simulink model "iface"  (R2018b)
settings: Solver=FixedStepDiscrete  StartTime=0.0  StopTime=10.0  RelTol=1e-3
settings Model: Creator=matlab  LastModifiedBy=matlab

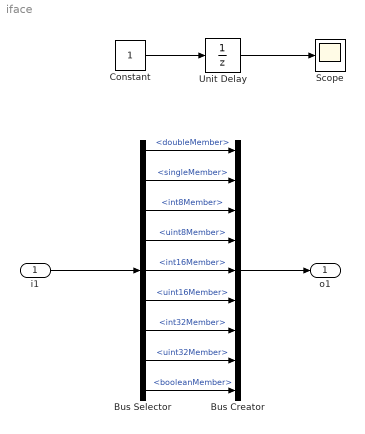
== system iface ==
  i1 : Inport  OutDataTypeStr=Bus: BusDef
  Bus Creator : BusCreator  Inputs=9  OutDataTypeStr=Bus: BusDef  NonVirtualBus=on
  Bus Selector : BusSelector  OutputSignals=doubleMember,singleMember,int8Member,uint8Member,int16Member,uint16Member,int32Member,uint32Member,booleanMember
  Constant : Constant
  Scope : Scope
  Unit Delay : UnitDelay  SampleTime=-1
  o1 : Outport  OutDataTypeStr=Bus: BusDef
  wires:
  Bus Creator/1 -> o1/1
  i1/1 -> Bus Selector/1
  Unit Delay/1 -> Scope/1
  Constant/1 -> Unit Delay/1
  Bus Selector/1 -> Bus Creator/1  "<doubleMember>"
  Bus Selector/2 -> Bus Creator/2  "<singleMember>"
  Bus Selector/3 -> Bus Creator/3  "<int8Member>"
  Bus Selector/4 -> Bus Creator/4  "<uint8Member>"
  Bus Selector/5 -> Bus Creator/5  "<int16Member>"
  Bus Selector/6 -> Bus Creator/6  "<uint16Member>"
  Bus Selector/7 -> Bus Creator/7  "<int32Member>"
  Bus Selector/8 -> Bus Creator/8  "<uint32Member>"
  Bus Selector/9 -> Bus Creator/9  "<booleanMember>"
